simulink subsystem "API221_GetError"  (R2022b)
settings: Solver=VariableStepAuto  StartTime=0.0  StopTime=10.0  RelTol=1e-3
settings Model: Creator=PROSTJP  LastModifiedBy=PROSTJP

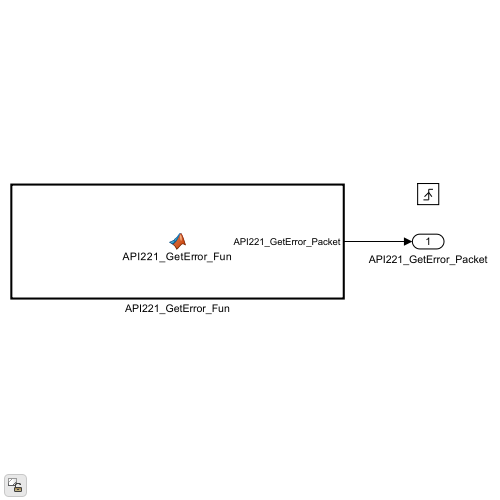
[thumbnail: Simulink's stored preview of the top-level diagram]
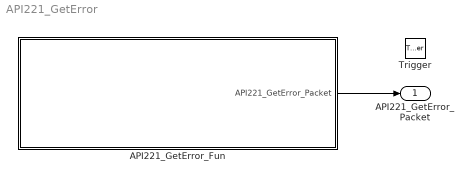
== system API221_GetError ==
  Trigger : TriggerPort  VariantControl=(inherit)  PortDimensions=1
  API221_GetError_Fun : MATLAB Function  TreatAsAtomicUnit=on
  API221_GetError_Packet : Outport
  wires:
  API221_GetError_Fun/1(API221_GetError_Packet) -> API221_GetError_Packet/1

== matlab function API221_GetError/API221_GetError_Fun ==
  data: API221_GetError_Packet output
function API221_GetError_Packet = API221_GetError_Fun()


    destination = 0;
    node_id = 1;
    sdu_length = 11;
    sap = 4;
    api_id = 221;
    op_code = 1;
    cmd_fb = 0;
    frag = 0;
    mmp = 0;

    destination_source = destination + node_id * (2^4);
    opcode_compl = op_code + cmd_fb * (2^5) + frag * (2^6) + mmp * (2^7);

    motor_idx = uint8(0);
    
    header_api221 = uint8([destination_source sap sdu_length api_id opcode_compl]);
    tmp = uint8([header_api221, motor_idx]);

    API221_GetError_Packet = zeros(100,1, 'uint8');
    API221_GetError_Packet(1:length(tmp)) = tmp;

end
